simulink model "cart_pend"  (R2019b)
settings: Solver=FixedStepAuto  StartTime=0.0  StopTime=10.0  FixedStep=0.01  RelTol=1e-3
settings Model: Creator=Murray  LastModifiedBy=Murray

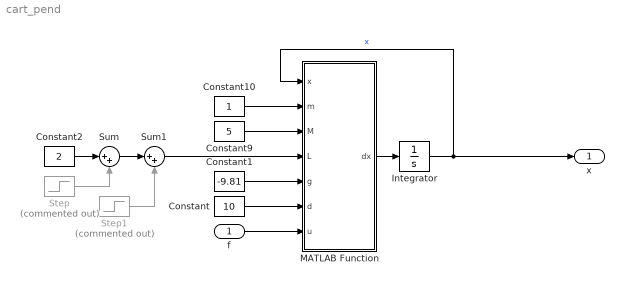
== system cart_pend ==
  f : Inport
  Constant : Constant  Value=10
  Constant1 : Constant  Value=-9.81
  Constant10 : Constant
  Constant2 : Constant  Value=2
  Constant9 : Constant  Value=5
  Integrator : Integrator  InitialCondition=[0; 0; 0; 0]
  MATLAB Function : MATLAB Function  TreatAsAtomicUnit=on
  Step : Step  Commented=on  Time=60  SampleTime=0
  Step1 : Step  Commented=on  Time=140  After=-2  SampleTime=0
  Sum : Sum  Inputs=|++
  Sum1 : Sum  Inputs=|++
  x : Outport
  wires:
  Constant9/1 -> MATLAB Function/3(M)
  Integrator/1 -> MATLAB Function/1(x), x/1  "x"
  Constant10/1 -> MATLAB Function/2(m)
  Constant1/1 -> MATLAB Function/5(g)
  MATLAB Function/1(dx) -> Integrator/1
  f/1 -> MATLAB Function/7(u)
  Constant/1 -> MATLAB Function/6(d)
  Constant2/1 -> Sum/1
  Step/1 -> Sum/2
  Sum/1 -> Sum1/1
  Sum1/1 -> MATLAB Function/4(L)
  Step1/1 -> Sum1/2

== matlab function cart_pend/MATLAB Function ==
  data: x input; m input; M input; L input; g input; d input; u input; dx output
function dx = cartpend(x,m,M,L,g,d,u)
%CARTPEND Models a continuous system of a pendulem on a cart.
%   based on Steve Brunton code. See youtube.com/watch?v=qjhAAQexzLg&list=PLMrJAkhIeNNR20Mz-VpzgfQs5zrYi085m&index=12
%   x  = state vector [x; x_dot; theta; theta_dot]
%   dx = derivative of state vector
%   u  = input vector [f]
%   m  = mass of pendulem end
%   M  = mass of cart
%   L  = length of pendulem rod
%   g  = acceleration due to gravity
%   d  = damping coef of friction on cart

Sx = sin(x(3));
Cx = cos(x(3));
D = m*L*L*(M+m*(1-Cx^2));

dx = zeros(4,1);

dx(1,1) = x(2);
dx(2,1) = (1/D)*(-m^2*L^2*g*Cx*Sx + m*L^2*(m*L*x(4)^2*Sx - d*x(2))) + m*L*L*(1/D)*u;
dx(3,1) = x(4);
dx(4,1) = (1/D)*((m+M)*m*g*L*Sx - m*L*Cx*(m*L*x(4)^2*Sx - d*x(2))) - m*L*Cx*(1/D)*u; % +.01*randn;
